simulink model "TWFL_V1"  (R2025b)
settings: Solver=daessc  StartTime=0.0  StopTime=20  RelTol=1e-3
undefined symbols (not defined in the file): dspblkCoreblockFVToolHelper, g, g_fork, g_lift, gcbh, Kd_fork, Kd_lift, Kp_fork, Kp_lift, lx, ly, lz, M, m_w, Mn_33, Mn_44, N, r, T_control, X, Y, Z
libraries: sm_lib x80, nesl_utility x21, simulink x5, slpidlib x1
(part 1 of 3)
settings Model: Creator=oj  LastModifiedBy=itsan
settings DataIOCC: SaveFormat=StructureWithTime
settings OptimizationCC: LifeSpan=inf
settings DebuggingCC: UnconnectedInputMsg=warning  UnconnectedOutputMsg=warning  UnconnectedLineMsg=warning  SFExecutionAtInitializationDiag=none  ArithmeticOperatorsInVariantConditions=warning
settings HardwareCC: ProdBitPerSizeT=32.0  ProdBitPerPtrDiffT=32.0  ProdWordSize=32.0  ProdHWDeviceType=Specified
settings SFSimCC: CustomCodeUndefinedFunction=UseInterfaceOnly
settings RTWCC: GPUComputeCapability=3.5
settings CodeAppCC: StateflowObjectComments=on

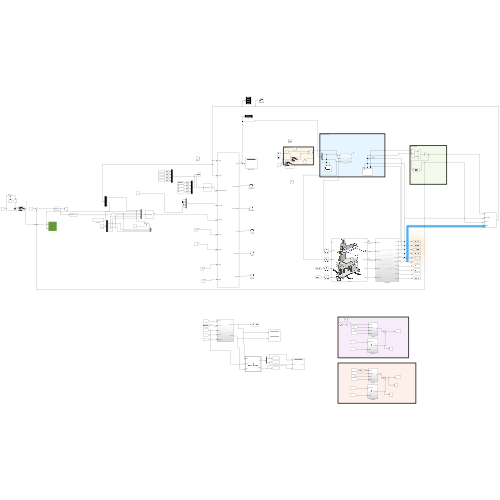
[thumbnail: Simulink's stored preview of the top-level diagram]
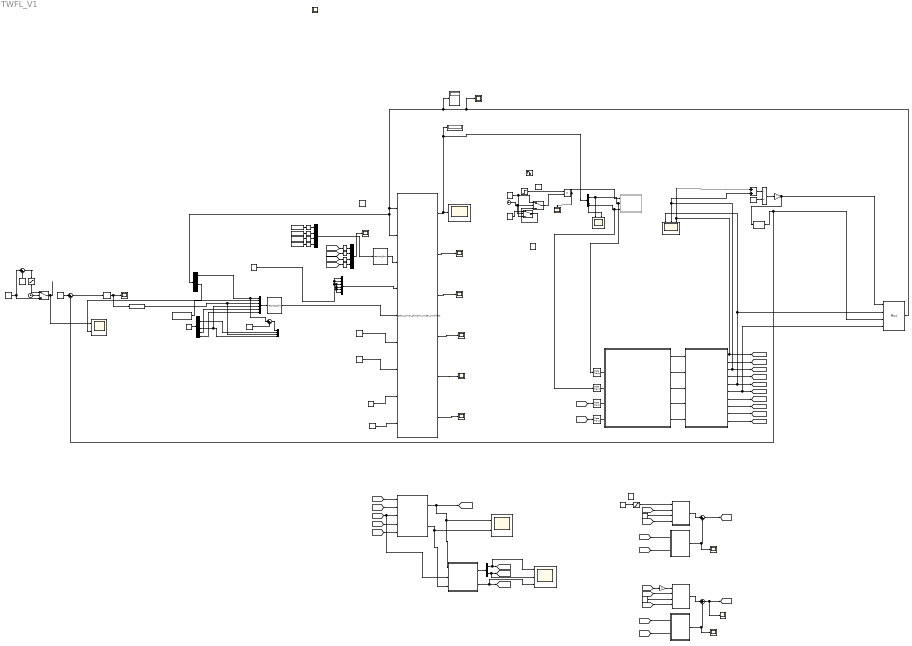
== system TWFL_V1 ==
  note: Simscape model
  note: Calculations
  note: Disturbance
  CPU : Scope
      settings: Description=status  ActiveDisplayYMinimum=-0.000978492283750898  ActiveDisplayYMaximum=0.0013917002145656821  DataLoggingVariableName=ScopeData3
  Calculations : Subsystem
  Clock : Clock
      settings: Decimation=7
  Clock1 : Clock
      settings: Decimation=9
  Constant{,8,13,42..43} (5 alike) : Constant  Value=0
  Constant1 : Constant
  Constant10 : Constant  Value=6
  Constant11 : Constant  Value=-0.1
  Constant12 : Constant  Value=0.8
  Constant14 : Constant  Value=2
  Constant15 : Constant
  Constant2 : Constant  Value=repmat([-50; -pi/4; -3; -pi],N-1,1)
  Constant3 : Constant  Value=repmat([-10;-10],N,1)
  Constant4 : Constant  Value=repmat([500; pi/4; 3; pi],N-1,1)
  Constant45 : Constant  Value=0.0
  Constant5 : Constant
  Constant6 : Constant  Value=2
  Constant7 : Constant  Value=repmat([10;10],N,1)
  Constant9 : Constant  Value=2
  Demux : Demux  Outputs=2
  Demux1 : Demux  Outputs=2
  Demux2 : Demux
  Demux3 : Demux  Outputs=6
  Discrete Derivative : simulink/Discrete/Discrete Derivative  gainval=1.0  ICPrevScaledInput=0.0  OutMin=[]  OutMax=[]  OutDataType=fixdt(1, 16)  OutScaling=2^-10  DoSatur=off
  Display1 : Display
  Divide : Product  Inputs=**
  Divide1 : Product  Inputs=*/
  Fork DOB : Subsystem
  Gain18 : Gain  Gain=-1
  Gain2 : Gain  Gain=r
  KKT residual : Scope
      settings: Description=status  ActiveDisplayYMinimum=-0.32883901659053916  ActiveDisplayYMaximum=1.592767698176573  DataLoggingVariableName=ScopeData4
  Lift DOB : Subsystem
  MATLAB Function1 : MATLAB Function  TreatAsAtomicUnit=on
  Mux{,1,4..5} (4 alike) : Mux
      Mux settings: DisplayOption=signals
  Mux2 : Mux  Inputs=6
  Mux3 : Mux  Inputs=6
  OCP status : Scope
      settings: Description=status  ActiveDisplayYMinimum=-2.0851401210050069  ActiveDisplayYMaximum=5.2280116787993132
  PD fork : Subsystem
  PD lift : Subsystem
  PID Controller : slpidlib/PID Controller  Controller=PID  Form=Parallel  TimeDomain=Discrete-time  UseExternalTs=off  SampleTime=-1  IntegratorMethod=Forward Euler  FilterMethod=Forward Euler  ControllerParametersSource=internal  P=2  I=1  UseKiTs=off  D=0  UseExternalDerivativeSource=off  N=100  UseFilter=on  TunerSelectOption=Transfer Function Based (PID Tuner App)  InitialConditionSource=internal  InitialConditionForIntegrator=0  InitialConditionForFilter=0  DifferentiatorICPrevScaledInput=0  ExternalReset=none  TrackingMode=off  Kt=1  LimitOutput=off  SatLimitsSource=internal  UpperSaturationLimit=inf  LowerSaturationLimit=-inf  LinearizeAsGain=on  AntiWindupMode=none  Kb=1  LimitIntegrator=off  UpperIntegratorSaturationLimit=inf  LowerIntegratorSaturationLimit=-inf  POutMin=[]  POutMax=[]  IOutMin=[]  IOutMax=[]  DOutMin=[]  DOutMax=[]  NOutMin=[]  NOutMax=[]  SumOutMin=[]  SumOutMax=[]  SaturationOutMin=[]  SaturationOutMax=[]  PParamMin=[]  PParamMax=[]  IParamMin=[]  IParamMax=[]  DParamMin=[]  DParamMax=[]  NParamMin=[]  NParamMax=[]  KbParamMin=[]  KbParamMax=[]  KtParamMin=[]  KtParamMax=[]  KbOutMin=[]  KbOutMax=[]  KtOutMin=[]  KtOutMax=[]  IntegratorOutMin=[]  IntegratorOutMax=[]  FilterOutMin=[]  FilterOutMax=[]  SumI1OutMin=[]  SumI1OutMax=[]  SumI2OutMin=[]  SumI2OutMax=[]  SumI3OutMin=[]  SumI3OutMax=[]  SumI4OutMin=[]  SumI4OutMax=[]  SumDOutMin=[]  SumDOutMax=[]  DifferentiatorOutMin=[]  DifferentiatorOutMax=[]  FilterDiffOutCoefMin=[]  FilterDiffOutCoefMax=[]  ReciprocalOutMin=[]  ReciprocalOutMax=[]  SumDenOutMin=[]  SumDenOutMax=[]  SumNumOutMin=[]  SumNumOutMax=[]  DivideOutMin=[]  DivideOutMax=[]  UdiffTsProdOutMin=[]  UdiffTsProdOutMax=[]  NTsProdOutMin=[]  NTsProdOutMax=[]  UintegralTsProdOutMin=[]  UintegralTsProdOutMax=[]  UngainTsProdOutMin=[]  UngainTsProdOutMax=[]  ClampingZeroOutDataTypeStr=Inherit: Inherit via back propagation  ClampingZeroOutMin=[]  ClampingZeroOutMax=[]  FilterDenConstantOutDataTypeStr=Inherit: Inherit via back propagation  FilterDenConstantOutMin=[]  FilterDenConstantOutMax=[]  PCopyOutDataTypeStr=Inherit: Inherit via back propagation  PCopyOutMin=[]  PCopyOutMax=[]  NCopyOutDataTypeStr=Inherit: Inherit via back propagation  NCopyOutMin=[]  NCopyOutMax=[]  IntegratorContinuousStateAttributes=''  IntegratorStateMustResolveToSignalObject=off  IntegratorRTWStateStorageClass=Auto  FilterContinuousStateAttributes=''  FilterStateMustResolveToSignalObject=off  FilterRTWStateStorageClass=Auto  ParallelPVariant=InternalParameters  IdealPVariant=Disabled  IVariant=InternalParameters  DVariant=InternalParameters  IntegratorVariant=Discrete  SatVariant=Disabled  AWVariant=Passthrough  PCopyVariant=Disabled  TRVariant=Disabled  FdbkBlocksVariant=Forward  IdealPFdbkVariant=Disabled  SatFdbkVariant=Disabled  DerivativeFilterVariant=ForwardEulerFilter  NVariant=InternalParameters  NCopyVariant=Disabled  FilterICVariant=InternalICsFilter  IntegratorICVariant=InternalICs  ExternalResetVariant=Disabled  TRSumVariant=Passthrough  SumFdbkVariant=Disabled  SumVariant=Sum_PID  TsampFilterVariant=InternalTs  TsampNgainVariant=Passthrough  TsampIntegralVariant=Disabled_SignalSpec  ExternalSaturationOutDataTypeStr=Inherit: Same as second input  DerivativeSourceVariant=ErrorSignal  PreIntVariant=InternalPreInt
  Plant : Subsystem  Commented=on
  Plant5 : Subsystem
      mask Display: image('plant.png');
  Ramp : simulink/Sources/Ramp  slope=4  start=1  InitialOutput=0
  Ramp1 : simulink/Sources/Ramp  slope=0.05  start=1  InitialOutput=0
  Ramp2 : simulink/Sources/Ramp  slope=1  start=9  InitialOutput=0
  Rate Transition{,1..3} (4 alike) : RateTransition  OutPortSampleTime=T_control
  S-Function : S-Function  FunctionName=repmat_sfun  Parameters=N-1  SFunctionDeploymentMode=off  EnableBusSupport=off
  S-Function1 : S-Function  FunctionName=acados_solver_sfunction_model_simplified  SFunctionDeploymentMode=off  EnableBusSupport=off
      mask Display:
      | % from the make_sfun file
      | global sfun_input_names sfun_output_names
      | for i = 1:length(sfun_input_names)
      | 	port_label('input', i, sfun_input_names{i})
      | end
      | for i = 1:length(sfun_output_names)
      | 	port_label('output', i, sfun_output_names{i})
      | end
  S-Function2 : S-Function  FunctionName=repmat_sfun  Parameters=N+1  SFunctionDeploymentMode=off  EnableBusSupport=off
  SQP iter : Scope
      settings: Description=status  ActiveDisplayYMinimum=0.875  ActiveDisplayYMaximum=2.125  DataLoggingVariableName=ScopeData5
  Saturation : Saturate  UpperLimit=5  LowerLimit=0
  Saturation2 : Saturate  UpperLimit=.25
  Scope control : Scope
      settings: ActiveDisplayYMinimum=-179.76344795838239  ActiveDisplayYMaximum=28.261944980460278  DataLoggingVariableName=ScopeData6
  Scope state : Scope
      settings: ActiveDisplayYMinimum=-0.50123790367694254  ActiveDisplayYMaximum=0.42460054813556447  DataLoggingVariableName=ScopeData7
  Scope2 : Scope  NumInputPorts=3
      settings: ActiveDisplayYMinimum=-0.20198063479091835  ActiveDisplayYMaximum=0.15327811856996762  DataLoggingVariableName=ScopeData9
  Scope26 : Scope  NumInputPorts=2
      settings: ActiveDisplayYMinimum=-5.5444382894798494  ActiveDisplayYMaximum=19.314835391492366  DataLoggingVariableName=ScopeData32
  Scope{,4..5,7,29..31} (7 alike) : Scope
      Scope29 settings: ActiveDisplayYMinimum=-96.648348177302324  ActiveDisplayYMaximum=-32.034536436658129  DataLoggingVariableName=ScopeData36
      Scope30 settings: ActiveDisplayYMinimum=-184.47481197821281  ActiveDisplayYMaximum=541.97444620327656  DataLoggingVariableName=ScopeData35
      Scope31 settings: ActiveDisplayYMinimum=-107.02501908705908  ActiveDisplayYMaximum=9.012103475779579  DataLoggingVariableName=ScopeData37
      Scope4 settings: ActiveDisplayYMinimum=-15.603117153759081  ActiveDisplayYMaximum=28.598103704711281  DataLoggingVariableName=ScopeData11
      Scope5 settings: ActiveDisplayYMinimum=-0.32762488910758569  ActiveDisplayYMaximum=3.4436733955388874  DataLoggingVariableName=ScopeData12
      Scope7 settings: ActiveDisplayYMinimum=-0.36432624038755357  ActiveDisplayYMaximum=6.747864665777934  DataLoggingVariableName=ScopeData19
      Scope settings: ActiveDisplayYMinimum=-13.79726  ActiveDisplayYMaximum=10.28583
  Scope3 : Scope  NumInputPorts=2
      settings: ActiveDisplayYMinimum=-0.28208251457945138  ActiveDisplayYMaximum=0.11496904410617963  DataLoggingVariableName=ScopeData10
  Scope6 : Scope  NumInputPorts=2
      settings: ActiveDisplayYMinimum=-1.0752841178040073  ActiveDisplayYMaximum=3.1865041498100037  DataLoggingVariableName=ScopeData13
  Scope8 : Scope  NumInputPorts=3
      settings: ActiveDisplayYMinimum=-5.0680991382670406  ActiveDisplayYMaximum=15.726284673069914  DataLoggingVariableName=ScopeData21
  Signal Specification : SignalSpecification  OutDataTypeStr=double  Dimensions=1
  Signal Specification{1..8} (8 alike) : SignalSpecification  Dimensions=1
  Sine Wave : Sin  Frequency=6*pi  SampleTime=0
  Step : Step  After=30  SampleTime=0
  Subsystem : Subsystem
  Sum : Sum  Inputs=+|+
  Sum16 : Sum  Inputs=|++
  Sum17 : Sum  Inputs=|++
  Sum3 : Sum  Inputs=|+-
  Sum4 : Sum  Inputs=|++
  Sum5 : Sum  Inputs=|+-
  Switch : Switch  Criteria=u2 > Threshold  Threshold=4  SaturateOnIntegerOverflow=off  InputSameDT=off
  Switch1 : Switch  Criteria=u2 > Threshold  Threshold=3  SaturateOnIntegerOverflow=off  InputSameDT=off
  Switch2 : Switch  Criteria=u2 > Threshold  SaturateOnIntegerOverflow=off  InputSameDT=off
  ref pitch : Constant  Value=0.0535
  u : Display
  weights : Constant  Value=repmat([5;3;0;1e-3], 244/4, 1)
  x1 ocp : Scope
      settings: Description=status  ActiveDisplayYMinimum=-2.6422889921421415  ActiveDisplayYMaximum=2.2266101006407979  DataLoggingVariableName=ScopeData2
  y_ref4 : Constant  Value=[1; 0; 0; 0; 0; 0]
  wires:
  S-Function1/5 -> CPU/1
  S-Function1/6 -> SQP iter/1
  S-Function1/3 -> KKT residual/1
  Mux/1 -> Display1/1, Demux2/1, S-Function1/2, S-Function1/1, Scope state/1  "x"
  S-Function1/4 -> x1 ocp/1
  S-Function1/2 -> OCP status/1
  Clock/1 -> Switch1/2, Switch/2
  Constant/1 -> Switch1/3, Switch/1
  Divide/1 -> Scope5/1, Plant/1(dF)
  Switch/1 -> Divide/2
  S-Function1/1 -> u/1, Demux/1, Scope control/1  "u"
  Switch1/1 -> Switch/3
  Constant1/1 -> Switch1/1
  Constant2/1 -> S-Function1/6
  Mux3/1 -> S-Function1/4
  Demux/1 -> Scope3/1, Rate Transition2/1, Plant/2(rwTorque)
  Calculations/1(rw_pos) -> Sum/1, Scope2/3, [rw_pos]  "rw_angle"
  Calculations/3(lw_pos) -> Sum/2, Scope2/2, [lw_pos]  "lw_angle"
  Calculations/5(pitch_pos) -> Mux/2, Scope2/1, [pitch_pos]  "pitch_angle"
  Sum/1 -> Divide1/1
  Constant6/1 -> Divide1/2
  Divide1/1 -> Gain2/1
  Gain2/1 -> Discrete Derivative/1, Mux/1  "x"
  Discrete Derivative/1 -> Mux/3, Sum3/2  "x_dot"
  Constant3/1 -> S-Function1/8
  Constant7/1 -> S-Function1/9
  Step/1 -> Divide/1
  Demux/2 -> Rate Transition3/1, Plant/3(lwTorque), Scope3/2
  S-Function/1 -> S-Function1/5
  Mux2/1 -> S-Function/1
  y_ref4/1 -> Demux3/1
  Demux3/4 -> Mux2/4, Mux1/4
  Demux3/6 -> Mux2/6
  Demux3/5 -> Mux2/5
  Demux2/1 -> Sum4/1, Mux2/1
  Sum3/1 -> PID Controller/1
  Constant13/1 -> Mux3/1, Mux3/2, Mux3/6, Mux3/5, Mux3/4, Mux3/3
  Constant14/1 -> Switch2/3, Sum5/1
  PID Controller/1 -> Signal Specification/1, Scope4/1
  Signal Specification/1 -> Mux2/3, Mux1/3
  Demux3/2 -> Mux1/2
  Sum4/1 -> Mux1/1
  Constant15/1 -> Sum4/2
  Constant4/1 -> S-Function1/7
  Ramp2/1 -> Sum5/2
  Clock1/1 -> Switch2/2
  Sum5/1 -> Saturation/1
  Saturation/1 -> Switch2/1
  Switch2/1 -> Scope6/1  "reference_v"
  Demux2/3 -> Scope6/2
  ref pitch/1 -> Mux2/2
  Calculations/4(lw_vel) -> [lw_vel]
  Calculations/9(arm_pos) -> [arm_pos]
  Calculations/8(lift_vel) -> [lift_vel]
  Plant5/5(armPos) -> Calculations/5(arm_angle)
  Plant5/4(lift_pos) -> Calculations/4(lift_height)
  Calculations/7(lift_pos) -> [lift_pos]
  Rate Transition1/1 -> Plant5/4(liftForce)
  [force_lift] -> Rate Transition1/1
  [arm_pos] -> Subsystem/4(arm_pos)
  Rate Transition/1 -> Plant5/5(armTorque)
  Plant5/3(pitch_angle) -> Calculations/3(pitch_angle)  "pitch_angle"
  Calculations/6(pitch_vel) -> Mux/4, [pitch_vel]
  Plant5/1(rw_angle) -> Calculations/1(rw_angle)  "rw_angle"
  [force_lift] -> Subsystem/1(force_lift)
  Plant5/2(lw_angle) -> Calculations/2(lw_angle)  "lw_angle"
  [lift_pos] -> MATLAB Function1/2(pos_lift), Subsystem/3(lift_pos)
  Subsystem/1(mass_hat) -> [mass_hat], MATLAB Function1/1(m_hat), Scope26/1
  Calculations/2(rw_vel) -> [rw_vel]
  [torque_arm] -> Subsystem/5(torque_arm)
  [pitch_pos] -> Subsystem/2(pitch_pos)
  Calculations/10(arm_vel) -> [arm_vel]
  [torque_arm] -> Rate Transition/1
  Rate Transition2/1 -> Plant5/2(rwTorque)
  Rate Transition3/1 -> Plant5/3(lwTorque)
  Constant8/1 -> Sum3/1
  MATLAB Function1/1(cdg) -> Demux1/1
  Demux1/1 -> Scope8/1, [cog_x]
  Demux1/2 -> Scope8/2, [cog_z]
  MATLAB Function1/2(I_total) -> Scope8/3, [inertia]
  [mass_hat] -> Signal Specification4/1
  [inertia] -> Signal Specification3/1
  [cog_x] -> Signal Specification2/1
  [cog_z] -> Signal Specification1/1
  Signal Specification1/1 -> Mux4/4
  Signal Specification2/1 -> Mux4/3
  Signal Specification3/1 -> Mux4/2
  Signal Specification4/1 -> Mux4/1
  Subsystem/2(dist_hat) -> MATLAB Function1/3(d_hat), Scope26/2
  Sum17/1 -> [force_lift]
  [pitch_pos] -> Gain18/1
  [lift_pos] -> PD lift/2(posMeas)
  [force_lift] -> Lift DOB/1(Input Torque)
  Constant42/1 -> PD fork/3(velRef)
  Constant43/1 -> PD lift/3(velRef)
  Fork DOB/1(Est_dis) -> Scope29/1, Sum16/2
  Lift DOB/1(Est_dis) -> Sum17/2, Scope30/1
  [lift_vel] -> PD lift/4(velMeas)
  [torque_arm] -> Fork DOB/1(Input Torque)
  Sum16/1 -> Scope31/1, [torque_arm]
  PD lift/1(out) -> Sum17/1
  Ramp1/1 -> Saturation2/1
  [arm_vel] -> Fork DOB/2(Velocity)
  PD fork/1(out) -> Sum16/1
  Gain18/1 -> PD fork/1(posRef)
  [arm_vel] -> PD fork/4(velMeas)
  [lift_vel] -> Lift DOB/2(Velocity)
  [arm_pos] -> PD fork/2(posMeas)
  Mux4/1 -> Scope7/1
  S-Function2/1 -> S-Function1/3
  Signal Specification8/1 -> Mux5/1
  Signal Specification7/1 -> Mux5/2
  Signal Specification6/1 -> Mux5/3
  Signal Specification5/1 -> Mux5/4
  Constant12/1 -> Signal Specification5/1
  Constant11/1 -> Signal Specification6/1
  Constant10/1 -> Signal Specification7/1
  Constant9/1 -> Signal Specification8/1
  Mux5/1 -> S-Function2/1
  Saturation2/1 -> PD lift/1(posRef)

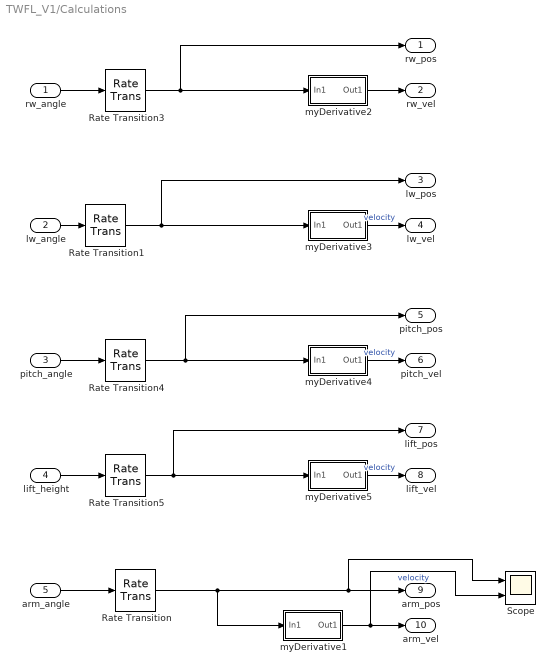
== system TWFL_V1/Calculations ==
  rw_angle : Inport
  lw_angle : Inport  Port=2
  pitch_angle : Inport  Port=3
  lift_height : Inport  Port=4
  arm_angle : Inport  Port=5
  Rate Transition{,1,3..5} (5 alike) : RateTransition  OutPortSampleTime=T_control
  Scope : Scope  NumInputPorts=2
      settings: ActiveDisplayYMinimum=-0.3840409140605956  ActiveDisplayYMaximum=2.1541582270060031  DataLoggingVariableName=ScopeData22
  myDerivative1 : Subsystem
      mask Display: image('myDerivative.png');
  myDerivative2 : Subsystem
      mask Display: image('myDerivative.png');
  myDerivative3 : Subsystem
      mask Display: image('myDerivative.png');
  myDerivative4 : Subsystem
      mask Display: image('myDerivative.png');
  myDerivative5 : Subsystem
      mask Display: image('myDerivative.png');
  rw_pos : Outport
  rw_vel : Outport  Port=2
  lw_pos : Outport  Port=3
  lw_vel : Outport  Port=4
  pitch_pos : Outport  Port=5
  pitch_vel : Outport  Port=6
  lift_pos : Outport  Port=7
  lift_vel : Outport  Port=8
  arm_pos : Outport  Port=9
  arm_vel : Outport  Port=10
  wires:
  rw_angle/1 -> Rate Transition3/1
  lw_angle/1 -> Rate Transition1/1
  pitch_angle/1 -> Rate Transition4/1
  Rate Transition5/1 -> myDerivative5/1(In1), lift_pos/1
  myDerivative2/1(Out1) -> rw_vel/1
  myDerivative3/1(Out1) -> lw_vel/1  "velocity"
  myDerivative4/1(Out1) -> pitch_vel/1  "velocity"
  myDerivative5/1(Out1) -> lift_vel/1  "velocity"
  lift_height/1 -> Rate Transition5/1
  arm_angle/1 -> Rate Transition/1
  myDerivative1/1(Out1) -> Scope/2, arm_vel/1  "velocity"
  Rate Transition/1 -> myDerivative1/1(In1), Scope/1, arm_pos/1
  Rate Transition1/1 -> myDerivative3/1(In1), lw_pos/1
  Rate Transition3/1 -> myDerivative2/1(In1), rw_pos/1
  Rate Transition4/1 -> myDerivative4/1(In1), pitch_pos/1

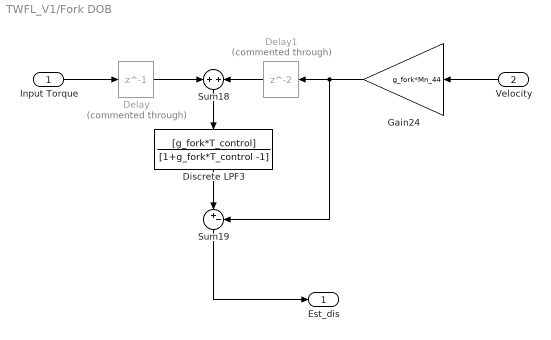
== system TWFL_V1/Fork DOB ==
  Input Torque : Inport
  Velocity : Inport  Port=2
  Delay : Delay  Commented=through  DelayLength=1  InputProcessing=Columns as channels (frame based)  SampleTime=T_control
  Delay1 : Delay  Commented=through  InputProcessing=Columns as channels (frame based)  SampleTime=T_control
  Discrete LPF3 : DiscreteFilter  LoadFcn=dspblkCoreblockFVToolHelper(gcbh,'load');  Numerator=[g_fork*T_control]  Denominator=[1+g_fork*T_control -1]
      settings: CopyFcn=dspblkCoreblockFVToolHelper(gcbh,'copy');  DeleteFcn=dspblkCoreblockFVToolHelper(gcbh,'close');  ModelCloseFcn=dspblkCoreblockFVToolHelper(gcbh,'close');  PreSaveFcn=dspblkCoreblockFVToolHelper(gcbh,'presave');  PostSaveFcn=dspblkCoreblockFVToolHelper(gcbh,'postsave');  CloseFcn=dspblkCoreblockFVToolHelper(gcbh,'close');
  Gain24 : Gain  Gain=g_fork*Mn_44
  Sum18 : Sum  Inputs=+|+
  Sum19 : Sum  Inputs=|+-
  Est_dis : Outport
  wires:
  Delay/1 -> Sum18/1
  Sum19/1 -> Est_dis/1
  Velocity/1 -> Gain24/1
  Input Torque/1 -> Delay/1
  Sum18/1 -> Discrete LPF3/1
  Gain24/1 -> Sum19/2, Delay1/1
  Discrete LPF3/1 -> Sum19/1
  Delay1/1 -> Sum18/2

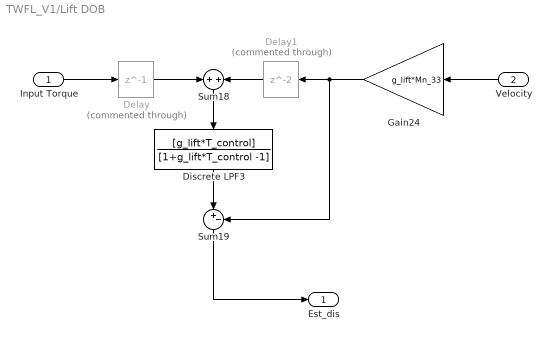
== system TWFL_V1/Lift DOB ==
  Input Torque : Inport
  Velocity : Inport  Port=2
  Delay : Delay  Commented=through  DelayLength=1  InputProcessing=Columns as channels (frame based)  SampleTime=T_control
  Delay1 : Delay  Commented=through  InputProcessing=Columns as channels (frame based)  SampleTime=T_control
  Discrete LPF3 : DiscreteFilter  LoadFcn=dspblkCoreblockFVToolHelper(gcbh,'load');  Numerator=[g_lift*T_control]  Denominator=[1+g_lift*T_control -1]
      settings: CopyFcn=dspblkCoreblockFVToolHelper(gcbh,'copy');  DeleteFcn=dspblkCoreblockFVToolHelper(gcbh,'close');  ModelCloseFcn=dspblkCoreblockFVToolHelper(gcbh,'close');  PreSaveFcn=dspblkCoreblockFVToolHelper(gcbh,'presave');  PostSaveFcn=dspblkCoreblockFVToolHelper(gcbh,'postsave');  CloseFcn=dspblkCoreblockFVToolHelper(gcbh,'close');
  Gain24 : Gain  Gain=g_lift*Mn_33
  Sum18 : Sum  Inputs=+|+
  Sum19 : Sum  Inputs=|+-
  Est_dis : Outport
  wires:
  Delay1/1 -> Sum18/2
  Discrete LPF3/1 -> Sum19/1
  Gain24/1 -> Delay1/1, Sum19/2
  Sum18/1 -> Discrete LPF3/1
  Input Torque/1 -> Delay/1
  Velocity/1 -> Gain24/1
  Sum19/1 -> Est_dis/1
  Delay/1 -> Sum18/1

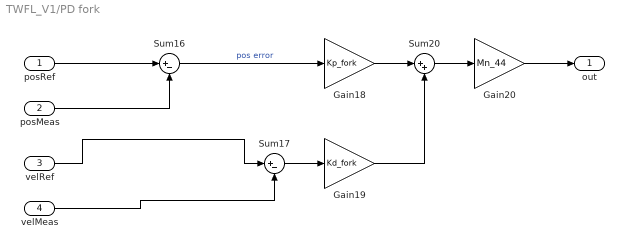
== system TWFL_V1/PD fork ==
  posRef : Inport
  posMeas : Inport  Port=2
  velRef : Inport  Port=3
  velMeas : Inport  Port=4
  Gain18 : Gain  Gain=Kp_fork
  Gain19 : Gain  Gain=Kd_fork
  Gain20 : Gain  Gain=Mn_44
  Sum16 : Sum  Inputs=|+-
  Sum17 : Sum  Inputs=|+-
  Sum20 : Sum  Inputs=|++
  out : Outport
  wires:
  Sum16/1 -> Gain18/1  "pos error"
  Gain18/1 -> Sum20/1
  Sum17/1 -> Gain19/1
  posRef/1 -> Sum16/1
  Sum20/1 -> Gain20/1
  Gain19/1 -> Sum20/2
  Gain20/1 -> out/1
  posMeas/1 -> Sum16/2
  velRef/1 -> Sum17/1
  velMeas/1 -> Sum17/2

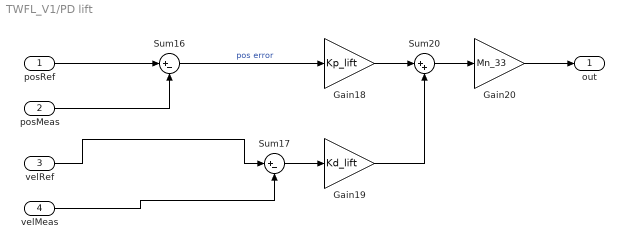
== system TWFL_V1/PD lift ==
  posRef : Inport
  posMeas : Inport  Port=2
  velRef : Inport  Port=3
  velMeas : Inport  Port=4
  Gain18 : Gain  Gain=Kp_lift
  Gain19 : Gain  Gain=Kd_lift
  Gain20 : Gain  Gain=Mn_33
  Sum16 : Sum  Inputs=|+-
  Sum17 : Sum  Inputs=|+-
  Sum20 : Sum  Inputs=|++
  out : Outport
  wires:
  velMeas/1 -> Sum17/2
  velRef/1 -> Sum17/1
  posMeas/1 -> Sum16/2
  Gain20/1 -> out/1
  Gain19/1 -> Sum20/2
  Sum20/1 -> Gain20/1
  posRef/1 -> Sum16/1
  Sum17/1 -> Gain19/1
  Gain18/1 -> Sum20/1
  Sum16/1 -> Gain18/1  "pos error"

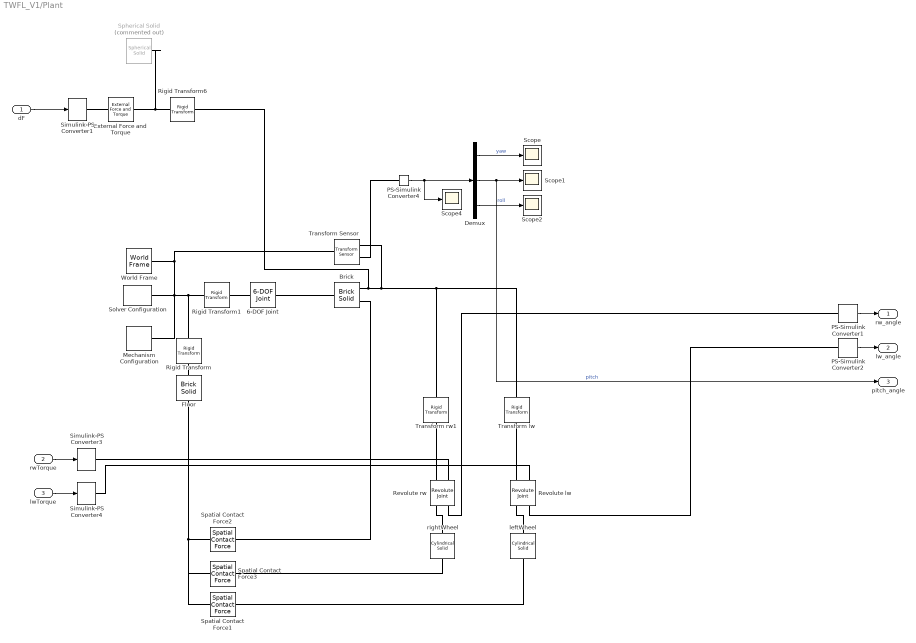
== system TWFL_V1/Plant ==
  dF : Inport
  rwTorque : Inport  Port=2
  lwTorque : Inport  Port=3
  6-DOF Joint : sm_lib/Joints/6-DOF Joint  JointMode=Normal  CompositeWrenchDir=BaseOnFollower  CompositeWrenchFrame=BaseFrame  SenseConstraintForce=off  SenseConstraintTorque=off  SenseTotalForce=off  SenseTotalTorque=off  PxPositionTargetSpecify=off  PxPositionTargetPriority=High  PxPositionTargetValue=0  PxPositionTargetValueUnits=m  PxVelocityTargetSpecify=off  PxVelocityTargetPriority=High  PxVelocityTargetValue=0  PxVelocityTargetValueUnits=m/s  PxEquilibriumPosition=0  PxEquilibriumPositionUnits=m  PxSpringStiffness=0  PxSpringStiffnessUnits=N/m  PxDampingCoefficient=0  PxDampingCoefficientUnits=N/(m/s)  PxLowerLimitSpecify=off  PxLowerLimitBound=-1  PxLowerLimitBoundUnits=m  PxLowerLimitStiffness=1e6  PxLowerLimitStiffnessUnits=N/m  PxLowerLimitDamping=1e3  PxLowerLimitDampingUnits=N/(m/s)  PxLowerLimitTransitionRegionWidth=1e-4  PxLowerLimitTransitionRegionWidthUnits=m  PxUpperLimitSpecify=off  PxUpperLimitBound=1  PxUpperLimitBoundUnits=m  PxUpperLimitStiffness=1e6  PxUpperLimitStiffnessUnits=N/m  PxUpperLimitDamping=1e3  PxUpperLimitDampingUnits=N/(m/s)  PxUpperLimitTransitionRegionWidth=1e-4  PxUpperLimitTransitionRegionWidthUnits=m  PxTorqueActuationMode=NoTorque  PxMotionActuationMode=ComputedMotion  PxSensePosition=off  PxSenseVelocity=off  PxSenseAcceleration=off  PxSenseTorqueForce=off  PxSenseLowerLimitTorqueForce=off  PxSenseUpperLimitTorqueForce=off  PyPositionTargetSpecify=off  PyPositionTargetPriority=High  PyPositionTargetValue=0  PyPositionTargetValueUnits=m  PyVelocityTargetSpecify=off  PyVelocityTargetPriority=High  PyVelocityTargetValue=0  PyVelocityTargetValueUnits=m/s  PyEquilibriumPosition=0  PyEquilibriumPositionUnits=m  PySpringStiffness=0  PySpringStiffnessUnits=N/m  PyDampingCoefficient=0  PyDampingCoefficientUnits=N/(m/s)  PyLowerLimitSpecify=off  PyLowerLimitBound=-1  PyLowerLimitBoundUnits=m  PyLowerLimitStiffness=1e6  PyLowerLimitStiffnessUnits=N/m  PyLowerLimitDamping=1e3  PyLowerLimitDampingUnits=N/(m/s)  PyLowerLimitTransitionRegionWidth=1e-4  PyLowerLimitTransitionRegionWidthUnits=m  PyUpperLimitSpecify=off  PyUpperLimitBound=1  PyUpperLimitBoundUnits=m  PyUpperLimitStiffness=1e6  PyUpperLimitStiffnessUnits=N/m  PyUpperLimitDamping=1e3  PyUpperLimitDampingUnits=N/(m/s)  PyUpperLimitTransitionRegionWidth=1e-4  PyUpperLimitTransitionRegionWidthUnits=m  PyTorqueActuationMode=NoTorque  PyMotionActuationMode=ComputedMotion  PySensePosition=off  PySenseVelocity=off  PySenseAcceleration=off  PySenseTorqueForce=off  PySenseLowerLimitTorqueForce=off  PySenseUpperLimitTorqueForce=off  PzPositionTargetSpecify=off  PzPositionTargetPriority=High  PzPositionTargetValue=0  PzPositionTargetValueUnits=m  PzVelocityTargetSpecify=off  PzVelocityTargetPriority=High  PzVelocityTargetValue=0  PzVelocityTargetValueUnits=m/s  PzEquilibriumPosition=0  PzEquilibriumPositionUnits=m  PzSpringStiffness=0  PzSpringStiffnessUnits=N/m  PzDampingCoefficient=0  PzDampingCoefficientUnits=N/(m/s)  PzLowerLimitSpecify=off  PzLowerLimitBound=-1  PzLowerLimitBoundUnits=m  PzLowerLimitStiffness=1e6  PzLowerLimitStiffnessUnits=N/m  PzLowerLimitDamping=1e3  PzLowerLimitDampingUnits=N/(m/s)  PzLowerLimitTransitionRegionWidth=1e-4  PzLowerLimitTransitionRegionWidthUnits=m  PzUpperLimitSpecify=off  PzUpperLimitBound=1  PzUpperLimitBoundUnits=m  PzUpperLimitStiffness=1e6  PzUpperLimitStiffnessUnits=N/m  PzUpperLimitDamping=1e3  PzUpperLimitDampingUnits=N/(m/s)  PzUpperLimitTransitionRegionWidth=1e-4  PzUpperLimitTransitionRegionWidthUnits=m  PzTorqueActuationMode=NoTorque  PzMotionActuationMode=ComputedMotion  PzSensePosition=off  PzSenseVelocity=off  PzSenseAcceleration=off  PzSenseTorqueForce=off  PzSenseLowerLimitTorqueForce=off  PzSenseUpperLimitTorqueForce=off  SphPositionTargetSpecify=off  SphPositionTargetPriority=High  SphPositionTargetRotationMethod=None  SphPositionTargetFollAlignAxisA=+X  SphPositionTargetBaseAlignAxisA=+Y  SphPositionTargetFollAlignAxisB=+Y  SphPositionTargetBaseAlignAxisB=+Z  SphPositionTargetRotationStandardAxis=+Z  SphPositionTargetRotationAngle=0  SphPositionTargetRotationAngleUnits=deg  SphPositionTargetRotationArbitraryAxis=[0 0 1]  SphPositionTargetRotationSequenceAxes=FollowerAxes  SphPositionTargetRotationSequence=XYX  SphPositionTargetRotationSequenceAngles=[0 0 0]  SphPositionTargetRotationSequenceAnglesUnits=deg  SphPositionTargetRotationMatrix=[1 0 0;0 1 0;0 0 1]  SphPositionTargetQuaternion=[1 0 0 0]  SphVelocityTargetSpecify=off  SphVelocityTargetPriority=High  SphVelocityTargetValue=[0 0 0]  SphVelocityTargetValueUnits=deg/s  SphVelocityTargetInFollowerFrame=on  SphEqPosRotationMethod=None  SphEqPosFollAlignAxisA=+X  SphEqPosBaseAlignAxisA=+Y  SphEqPosFollAlignAxisB=+Y  SphEqPosBaseAlignAxisB=+Z  SphEqPosRotationStandardAxis=+Z  SphEqPosRotationAngle=0  SphEqPosRotationAngleUnits=deg  SphEqPosRotationArbitraryAxis=[0 0 1]  SphEqPosRotationSequenceAxes=FollowerAxes  SphEqPosRotationSequence=XYX  SphEqPosRotationSequenceAngles=[0 0 0]  SphEqPosRotationSequenceAnglesUnits=deg  SphEqPosRotationMatrix=[1 0 0;0 1 0;0 0 1]  SphEqPosQuaternion=[1 0 0 0]  SphSpringStiffness=0  SphSpringStiffnessUnits=N*m/deg  SphDampingCoefficient=0  SphDampingCoefficientUnits=N*m/(deg/s)  SphLowerLimitSpecify=off  SphLowerLimitBound=15  SphLowerLimitBoundUnits=deg  SphLowerLimitStiffness=1e4  SphLowerLimitStiffnessUnits=N*m/deg  SphLowerLimitDamping=10  SphLowerLimitDampingUnits=N*m/(deg/s)  SphLowerLimitTransitionRegionWidth=0.1  SphLowerLimitTransitionRegionWidthUnits=deg  SphUpperLimitSpecify=off  SphUpperLimitBound=45  SphUpperLimitBoundUnits=deg  SphUpperLimitStiffness=1e4  SphUpperLimitStiffnessUnits=N*m/deg  SphUpperLimitDamping=10  SphUpperLimitDampingUnits=N*m/(deg/s)  SphUpperLimitTransitionRegionWidth=0.1  SphUpperLimitTransitionRegionWidthUnits=deg  SphTorqueActuationMode=NoTorque  SphActuateTorqueX=off  SphActuateTorqueY=off  SphActuateTorqueZ=off  SphActuateTorque=off  SphActuationFrame=BaseFrame  SphSensePosition=off  SphSenseVelocityX=off  SphSenseVelocityY=off  SphSenseVelocityZ=off  SphSenseVelocity=off  SphSenseAccelerationX=off  SphSenseAccelerationY=off  SphSenseAccelerationZ=off  SphSenseAcceleration=off  SphSenseLowerLimitTorqueMag=off  SphSenseUpperLimitTorqueMag=off  SphSensingFrame=BaseFrame
  Brick : sm_lib/Body Elements/Brick Solid  BrickDimensions=[lx ly lz]  BrickDimensionsUnits=m  ExportEntireGeometry=on  InertiaType=CalculateFromGeometry  BasedOnType=Mass  Density=1000  DensityUnits=kg/(m^3)  Mass=M  MassUnits=kg  CenterOfMass=[0 0 0]  CenterOfMassUnits=m  MomentsOfInertia=[1 1 1]  MomentsOfInertiaUnits=kg*m^2  ProductsOfInertia=[0 0 0]  ProductsOfInertiaUnits=kg*m^2  GraphicType=FromGeometry  MarkerShape=Sphere  MarkerSize=10  GraphicVisPropType=SimpleVisualProperties  GraphicDiffuseColor=[0.8 0.0 0.2]  GraphicOpacity=0.6  GraphicSpecularColor=[0.5 0.5 0.5 1.0]  GraphicAmbientColor=[0.15 0.15 0.15 1.0]  GraphicEmissiveColor=[0.0 0.0 0.0 1.0]  GraphicShininess=75  DoExposeReferenceFrame=on  SerializedFrames=|
      | <Frames>
      | 
      |   <Frame>
      |     <Id>Frame2</Id>
      |     <Value>
      |       <Name>B</Name>
      |       <Origin>
      |         <Source>GeometricFeature</Source>
      |         <FeatureName>-z surface</FeatureName>
      |       </Origin>
      |       <PrimaryAxis>
      |         <DefinedDirection>+Z</DefinedDirection>
      |         <Source>ReferenceFrame</Source>
      |         <SourceDirection>+Z</SourceDirection>
      |         <FeatureName></FeatureName>
      |       </PrimaryAxis>
      |       <SecondaryAxis>
      |         <DefinedDirection>+X</DefinedDirection>
      |         <Source>ReferenceFrame</Source>
      |         <SourceDirection>+X</SourceDirection>
      |         <FeatureName></FeatureName>
      |       </SecondaryAxis>
      |     </Value>
      |   </Frame>
      | 
      | </Frames>
  Demux : Demux  Outputs=3
  External Force and Torque : sm_lib/Forces and Torques/External Force and Torque  EnableForceX=on  EnableForceY=off  EnableForceZ=off  EnableForce=off  ForceResolutionFrame=World  EnableTorqueX=off  EnableTorqueY=off  EnableTorqueZ=off  EnableTorque=off  TorqueResolutionFrame=AttachedFrame
  Floor : sm_lib/Body Elements/Brick Solid  BrickDimensions=[100 100 0.010]  BrickDimensionsUnits=m  ExportEntireGeometry=on  InertiaType=CalculateFromGeometry  BasedOnType=Density  Density=1000  DensityUnits=kg/m^3  Mass=1  MassUnits=kg  CenterOfMass=[0 0 0]  CenterOfMassUnits=m  MomentsOfInertia=[1 1 1]  MomentsOfInertiaUnits=kg*m^2  ProductsOfInertia=[0 0 0]  ProductsOfInertiaUnits=kg*m^2  GraphicType=FromGeometry  MarkerShape=Sphere  MarkerSize=10  GraphicVisPropType=SimpleVisualProperties  GraphicDiffuseColor=[0.298 0.502 0.1294]  GraphicOpacity=1  GraphicSpecularColor=[0.5 0.5 0.5 1.0]  GraphicAmbientColor=[0.15 0.15 0.15 1.0]  GraphicEmissiveColor=[0.0 0.0 0.0 1.0]  GraphicShininess=75  DoExposeReferenceFrame=on  SerializedFrames=<Frames/>
  Mechanism Configuration : sm_lib/Utilities/Mechanism Configuration  UniformGravity=Constant  GravityVector=[0 0 -9.81]  GravityVectorUnits=m/s^2  LinearizationDelta=0.001  JointModeTransitionNonlinearIterations=2
  PS-Simulink Converter1 : nesl_utility/PS-Simulink Converter  PhysicalDomain=network_engine_domain  SubClassName=ps_output  LeftPortType=input  RightPortType=output  PseudoPeriodic=off  Frequencies=[]  VectorFormat=1-D array  Unit=1  AffineConversion=off
  PS-Simulink Converter2 : nesl_utility/PS-Simulink Converter  PhysicalDomain=network_engine_domain  SubClassName=ps_output  LeftPortType=input  RightPortType=output  PseudoPeriodic=off  Frequencies=[]  VectorFormat=1-D array  Unit=1  AffineConversion=off
  PS-Simulink Converter4 : nesl_utility/PS-Simulink Converter  PhysicalDomain=network_engine_domain  SubClassName=ps_output  LeftPortType=input  RightPortType=output  PseudoPeriodic=off  Frequencies=[]  VectorFormat=inherit  Unit=inherit  AffineConversion=off
  Revolute lw : sm_lib/Joints/Revolute Joint  JointMode=Normal  CompositeWrenchDir=FollowerOnBase  CompositeWrenchFrame=BaseFrame  SenseConstraintForce=off  SenseConstraintTorque=off  SenseTotalForce=off  SenseTotalTorque=off  PositionTargetSpecify=off  PositionTargetPriority=High  PositionTargetValue=0  PositionTargetValueUnits=deg  VelocityTargetSpecify=off  VelocityTargetPriority=High  VelocityTargetValue=0  VelocityTargetValueUnits=deg/s  EquilibriumPosition=0  EquilibriumPositionUnits=deg  SpringStiffness=0  SpringStiffnessUnits=N*m/deg  DampingCoefficient=0  DampingCoefficientUnits=N*m/(deg/s)  LowerLimitSpecify=off  LowerLimitBound=-90  LowerLimitBoundUnits=deg  LowerLimitStiffness=1e4  LowerLimitStiffnessUnits=N*m/deg  LowerLimitDamping=10  LowerLimitDampingUnits=N*m/(deg/s)  LowerLimitTransitionRegionWidth=0.1  LowerLimitTransitionRegionWidthUnits=deg  UpperLimitSpecify=off  UpperLimitBound=90  UpperLimitBoundUnits=deg  UpperLimitStiffness=1e4  UpperLimitStiffnessUnits=N*m/deg  UpperLimitDamping=10  UpperLimitDampingUnits=N*m/(deg/s)  UpperLimitTransitionRegionWidth=0.1  UpperLimitTransitionRegionWidthUnits=deg  TorqueActuationMode=InputTorque  MotionActuationMode=ComputedMotion  SensePosition=on  SenseVelocity=off  SenseAcceleration=off  SenseTorqueForce=off  SenseLowerLimitTorqueForce=off  SenseUpperLimitTorqueForce=off
  Revolute rw : sm_lib/Joints/Revolute Joint  JointMode=Normal  CompositeWrenchDir=FollowerOnBase  CompositeWrenchFrame=BaseFrame  SenseConstraintForce=off  SenseConstraintTorque=off  SenseTotalForce=off  SenseTotalTorque=off  PositionTargetSpecify=off  PositionTargetPriority=High  PositionTargetValue=0  PositionTargetValueUnits=deg  VelocityTargetSpecify=off  VelocityTargetPriority=High  VelocityTargetValue=0  VelocityTargetValueUnits=deg/s  EquilibriumPosition=0  EquilibriumPositionUnits=deg  SpringStiffness=0  SpringStiffnessUnits=N*m/deg  DampingCoefficient=0  DampingCoefficientUnits=N*m/(deg/s)  LowerLimitSpecify=off  LowerLimitBound=-90  LowerLimitBoundUnits=deg  LowerLimitStiffness=1e4  LowerLimitStiffnessUnits=N*m/deg  LowerLimitDamping=10  LowerLimitDampingUnits=N*m/(deg/s)  LowerLimitTransitionRegionWidth=0.1  LowerLimitTransitionRegionWidthUnits=deg  UpperLimitSpecify=off  UpperLimitBound=90  UpperLimitBoundUnits=deg  UpperLimitStiffness=1e4  UpperLimitStiffnessUnits=N*m/deg  UpperLimitDamping=10  UpperLimitDampingUnits=N*m/(deg/s)  UpperLimitTransitionRegionWidth=0.1  UpperLimitTransitionRegionWidthUnits=deg  TorqueActuationMode=InputTorque  MotionActuationMode=ComputedMotion  SensePosition=on  SenseVelocity=off  SenseAcceleration=off  SenseTorqueForce=off  SenseLowerLimitTorqueForce=off  SenseUpperLimitTorqueForce=off
  Rigid Transform : sm_lib/Frames and Transforms/Rigid Transform  RotationMethod=None  FollAlignAxisA=+X  BaseAlignAxisA=+Y  FollAlignAxisB=+Y  BaseAlignAxisB=+Z  RotationStandardAxis=+Z  RotationAngle=0  RotationAngleUnits=deg  RotationArbitraryAxis=[0 0 1]  RotationSequenceAxes=FollowerAxes  RotationSequence=XYX  RotationSequenceAngles=[0 0 0]  RotationSequenceAnglesUnits=deg  RotationMatrix=[1 0 0;0 1 0;0 0 1]  Quaternion=[1 0 0 0]  TranslationMethod=StandardAxis  TranslationCartesianOffset=[0 0 0]  TranslationCartesianOffsetUnits=m  TranslationStandardAxis=-Z  TranslationStandardOffset=0.005  TranslationStandardOffsetUnits=m  TranslationROffset=0  TranslationROffsetUnits=m  TranslationThetaOffset=0  TranslationThetaOffsetUnits=deg  TranslationZOffset=0  TranslationZOffsetUnits=m
  Rigid Transform1 : sm_lib/Frames and Transforms/Rigid Transform  RotationMethod=None  FollAlignAxisA=+X  BaseAlignAxisA=+Y  FollAlignAxisB=+Y  BaseAlignAxisB=+Z  RotationStandardAxis=+Z  RotationAngle=0  RotationAngleUnits=deg  RotationArbitraryAxis=[0 0 1]  RotationSequenceAxes=FollowerAxes  RotationSequence=XYX  RotationSequenceAngles=[0 0 0]  RotationSequenceAnglesUnits=deg  RotationMatrix=[1 0 0;0 1 0;0 0 1]  Quaternion=[1 0 0 0]  TranslationMethod=StandardAxis  TranslationCartesianOffset=[0 0 0]  TranslationCartesianOffsetUnits=m  TranslationStandardAxis=+Z  TranslationStandardOffset=0.5+0.2  TranslationStandardOffsetUnits=m  TranslationROffset=0  TranslationROffsetUnits=m  TranslationThetaOffset=0  TranslationThetaOffsetUnits=deg  TranslationZOffset=0  TranslationZOffsetUnits=m
  Rigid Transform6 : sm_lib/Frames and Transforms/Rigid Transform  RotationMethod=None  FollAlignAxisA=+X  BaseAlignAxisA=+Y  FollAlignAxisB=+Y  BaseAlignAxisB=+Z  RotationStandardAxis=+Y  RotationAngle=90  RotationAngleUnits=deg  RotationArbitraryAxis=[0 0 1]  RotationSequenceAxes=FollowerAxes  RotationSequence=XYX  RotationSequenceAngles=[0 0 0]  RotationSequenceAnglesUnits=deg  RotationMatrix=[0 0 1; 0 1 0; 1 0 0]  Quaternion=[1 0 0 0]  TranslationMethod=StandardAxis  TranslationCartesianOffset=[0 0 0]  TranslationCartesianOffsetUnits=m  TranslationStandardAxis=+Z  TranslationStandardOffset=1  TranslationStandardOffsetUnits=m  TranslationROffset=0  TranslationROffsetUnits=m  TranslationThetaOffset=0  TranslationThetaOffsetUnits=deg  TranslationZOffset=0  TranslationZOffsetUnits=m
  Scope{,1..2,4} (4 alike) : Scope
      Scope settings: ActiveDisplayYMinimum=-2.0138256178390441  ActiveDisplayYMaximum=0.22375840215241163  DataLoggingVariableName=ScopeData14
      Scope1 settings: ActiveDisplayYMinimum=-1.7669526132397224  ActiveDisplayYMaximum=0.19632806813774689  DataLoggingVariableName=ScopeData15
      Scope2 settings: ActiveDisplayYMinimum=-1  ActiveDisplayYMaximum=1  DataLoggingVariableName=ScopeData16
      Scope4 settings: ActiveDisplayYMinimum=-3.5002430122464903  ActiveDisplayYMaximum=3.7161890846826382  DataLoggingVariableName=ScopeData18
  Simulink-PS Converter1 : nesl_utility/Simulink-PS Converter  PhysicalDomain=network_engine_domain  SubClassName=ps_input  LeftPortType=input  RightPortType=output  PseudoPeriodic=off  Frequencies=[]  NoiseDistribution=none  NoiseParameters=[]  Unit=1  AffineConversion=off  FilteringAndDerivatives=zero  SimscapeFilterOrder=1  InputFilterTimeConstant=0.001  UdotUserProvided=1
  Simulink-PS Converter3 : nesl_utility/Simulink-PS Converter  PhysicalDomain=network_engine_domain  SubClassName=ps_input  LeftPortType=input  RightPortType=output  PseudoPeriodic=off  Frequencies=[]  NoiseDistribution=none  NoiseParameters=[]  Unit=1  AffineConversion=off  FilteringAndDerivatives=zero  SimscapeFilterOrder=1  InputFilterTimeConstant=0.001  UdotUserProvided=1
  Simulink-PS Converter4 : nesl_utility/Simulink-PS Converter  PhysicalDomain=network_engine_domain  SubClassName=ps_input  LeftPortType=input  RightPortType=output  PseudoPeriodic=off  Frequencies=[]  NoiseDistribution=none  NoiseParameters=[]  Unit=1  AffineConversion=off  FilteringAndDerivatives=zero  SimscapeFilterOrder=1  InputFilterTimeConstant=0.001  UdotUserProvided=1
  Solver Configuration : nesl_utility/Solver Configuration  PhysicalDomain=network_engine_domain  SubClassName=solver  LeftPortType=input  RightPortType=generic  Tones=[]  Harmonics=[]  SimulateNoise=off  Profile=off  UseLocalSampling=off  EnableSwitchedLinearOptims=on  FrequencyDomain=off  UseCCode=off  RelTol=0.001  AbsTol=1e-06  MinStep=1e-09  ToWorkspace=off  RevertToSquareIcSolve=off  NumHomotopyIterations=100  PhasorMode=off  PhasorModeNumHarmonics=1  ConsistencySolver=NEWTON_FTOL  IndexReductionMethod=DerivativeReplacement  DoDC=off  ResidualTolerance=1e-09  ConsistencyTolSource=GLOBAL  ConsistencyAbsTol=0.001  ConsistencyRelTol=0.001  ConsistencyTolFactor=0.001  UseLocalSolver=off  LocalSolverChoice=NE_BACKWARD_EULER_ADVANCER  ResolveIndetEquations=on  FunctionEvalNumThread=1  LocalSolverSampleTime=0.001  DoFixedCost=off  MaxNonlinIter=3  MaxModeIter=2  ComputeImpulses=off  ImpulseIterations=2  LinearAlgebra=Sparse  LinearAlgebraNumThread=0  EquationFormulation=NE_TIME_EF  DelaysMemoryBudget=1024  AutomaticFiltering=on  FilteringTimeConstant=0.001  PartitionStorageMethod=AS_NEEDED  PartitionMemoryBudget=1024  PartitionMethod=FAST  MultibodyUseLocalSolver=off  MultibodyLocalSolverChoice=ODE1  MultibodyLocalSolverSampleTime=0.001
  Spatial Contact Force1 : sm_lib/Forces and Torques/Spatial Contact Force  SenseSeparationDistance=off  NormalForceType=SmoothSpringDamper  NormalStiffness=1e6  NormalStiffnessUnits=N/m  NormalDamping=1e3  NormalDampingUnits=N/(m/s)  NormalTransitionRegionWidth=1e-4  NormalTransitionRegionWidthUnits=m  FrictionType=SmoothStickSlip  CoefficientOfStaticFriction=1  CoefficientOfDynamicFriction=1  FrictionalCriticalVelocity=1  FrictionalCriticalVelocityUnits=m/s  SenseContactSignal=off  SensePenetrationDepth=off  SenseNormalVelocity=off  SenseTangentialVelocity=off  SensingForceTorqueDirection=BaseOnFollower  SensingForceTorqueResolutionFrame=ContactFrame  SenseNormalForce=off  SenseNormalForceMagnitude=off  SenseNormalTorque=off  SenseFrictionalForce=off  SenseFrictionalForceMagnitude=off  SenseFrictionalTorque=off  SenseTotalForce=off  SenseTotalTorque=off  SenseContactBaseRotation=off  SenseContactBaseTranslation=off  SenseContactFollowerRotation=off  SenseContactFollowerTranslation=off  ZeroCrossDetectContactStartAndEnd=off
  Spatial Contact Force2 : sm_lib/Forces and Torques/Spatial Contact Force  SenseSeparationDistance=off  NormalForceType=SmoothSpringDamper  NormalStiffness=1e6  NormalStiffnessUnits=N/m  NormalDamping=1e3  NormalDampingUnits=N/(m/s)  NormalTransitionRegionWidth=1e-4  NormalTransitionRegionWidthUnits=m  FrictionType=SmoothStickSlip  CoefficientOfStaticFriction=0.5  CoefficientOfDynamicFriction=0.3  FrictionalCriticalVelocity=1e-3  FrictionalCriticalVelocityUnits=m/s  SenseContactSignal=off  SensePenetrationDepth=off  SenseNormalVelocity=off  SenseTangentialVelocity=off  SensingForceTorqueDirection=BaseOnFollower  SensingForceTorqueResolutionFrame=ContactFrame  SenseNormalForce=off  SenseNormalForceMagnitude=off  SenseNormalTorque=off  SenseFrictionalForce=off  SenseFrictionalForceMagnitude=off  SenseFrictionalTorque=off  SenseTotalForce=off  SenseTotalTorque=off  SenseContactBaseRotation=off  SenseContactBaseTranslation=off  SenseContactFollowerRotation=off  SenseContactFollowerTranslation=off  ZeroCrossDetectContactStartAndEnd=off
  Spatial Contact Force3 : sm_lib/Forces and Torques/Spatial Contact Force  SenseSeparationDistance=off  NormalForceType=SmoothSpringDamper  NormalStiffness=1e6  NormalStiffnessUnits=N/m  NormalDamping=1e3  NormalDampingUnits=N/(m/s)  NormalTransitionRegionWidth=1e-4  NormalTransitionRegionWidthUnits=m  FrictionType=SmoothStickSlip  CoefficientOfStaticFriction=1  CoefficientOfDynamicFriction=1  FrictionalCriticalVelocity=1  FrictionalCriticalVelocityUnits=m/s  SenseContactSignal=off  SensePenetrationDepth=off  SenseNormalVelocity=off  SenseTangentialVelocity=off  SensingForceTorqueDirection=BaseOnFollower  SensingForceTorqueResolutionFrame=ContactFrame  SenseNormalForce=off  SenseNormalForceMagnitude=off  SenseNormalTorque=off  SenseFrictionalForce=off  SenseFrictionalForceMagnitude=off  SenseFrictionalTorque=off  SenseTotalForce=off  SenseTotalTorque=off  SenseContactBaseRotation=off  SenseContactBaseTranslation=off  SenseContactFollowerRotation=off  SenseContactFollowerTranslation=off  ZeroCrossDetectContactStartAndEnd=off
  Spherical Solid : sm_lib/Body Elements/Spherical Solid  Commented=on  SphereRadius=0.1  SphereRadiusUnits=m  ExportEntireGeometry=off  InertiaType=CalculateFromGeometry  BasedOnType=Density  Density=1000  DensityUnits=kg/m^3  Mass=6  MassUnits=kg  CenterOfMass=[0 0 0]  CenterOfMassUnits=m  MomentsOfInertia=[1 1 1]  MomentsOfInertiaUnits=kg*m^2  ProductsOfInertia=[0 0 0]  ProductsOfInertiaUnits=kg*m^2  GraphicType=FromGeometry  MarkerShape=Sphere  MarkerSize=10  GraphicVisPropType=AdvancedVisualProperties  GraphicDiffuseColor=[0.5 0.5 0.5]  GraphicOpacity=1  GraphicSpecularColor=[0.8275 0.8275 0.8275]  GraphicAmbientColor=[0.15 0.15 0.15 1.0]  GraphicEmissiveColor=[0.0 0.0 0.0 1.0]  GraphicShininess=75  DoExposeReferenceFrame=on  SerializedFrames=<Frames/>
  Transform Sensor : sm_lib/Frames and Transforms/Transform Sensor  MeasurementFrame=World  RotationSequence=ZYX  SenseAngle=off  SenseAxis=off  SenseQ=off  SenseR=off  SenseRotationSequence=on  SenseOmegaX=off  SenseOmegaY=off  SenseOmegaZ=off  SenseOmega=off  SenseQDot=off  SenseRDot=off  SenseRotationSequenceDot=off  SenseAlphaX=off  SenseAlphaY=off  SenseAlphaZ=off  SenseAlpha=off  SenseQDDot=off  SenseRDDot=off  SenseX=off  SenseY=off  SenseZ=off  SenseXYZ=off  SenseRad=off  SenseAzim=off  SenseDist=off  SenseInc=off  SenseXDot=off  SenseYDot=off  SenseZDot=off  SenseXYZDot=off  SenseRadDot=off  SenseAzimDot=off  SenseDistDot=off  SenseIncDot=off  SenseXDDot=off  SenseYDDot=off  SenseZDDot=off  SenseXYZDDot=off  SenseRadDDot=off  SenseAzimDDot=off  SenseDistDDot=off  SenseIncDDot=off
  Transform lw : sm_lib/Frames and Transforms/Rigid Transform  RotationMethod=StandardAxis  FollAlignAxisA=+X  BaseAlignAxisA=+Y  FollAlignAxisB=+Y  BaseAlignAxisB=+Z  RotationStandardAxis=-X  RotationAngle=90  RotationAngleUnits=deg  RotationArbitraryAxis=[0 0 1]  RotationSequenceAxes=FollowerAxes  RotationSequence=XYX  RotationSequenceAngles=[0 0 0]  RotationSequenceAnglesUnits=deg  RotationMatrix=[1 0 0; 0 1 0; 0 0 1]  Quaternion=[1 0 0 0]  TranslationMethod=StandardAxis  TranslationCartesianOffset=[0 0 0]  TranslationCartesianOffsetUnits=m  TranslationStandardAxis=+Y  TranslationStandardOffset=ly/2+t/2  TranslationStandardOffsetUnits=m  TranslationROffset=0  TranslationROffsetUnits=m  TranslationThetaOffset=0  TranslationThetaOffsetUnits=deg  TranslationZOffset=0  TranslationZOffsetUnits=m
  Transform rw1 : sm_lib/Frames and Transforms/Rigid Transform  RotationMethod=StandardAxis  FollAlignAxisA=+X  BaseAlignAxisA=+Y  FollAlignAxisB=+Y  BaseAlignAxisB=+Z  RotationStandardAxis=-X  RotationAngle=90  RotationAngleUnits=deg  RotationArbitraryAxis=[0 0 1]  RotationSequenceAxes=FollowerAxes  RotationSequence=XYX  RotationSequenceAngles=[0 0 0]  RotationSequenceAnglesUnits=deg  RotationMatrix=[1 0 0; 0 1 0; 0 0 1]  Quaternion=[1 0 0 0]  TranslationMethod=StandardAxis  TranslationCartesianOffset=[0 0 0]  TranslationCartesianOffsetUnits=m  TranslationStandardAxis=-Y  TranslationStandardOffset=ly/2+t/2  TranslationStandardOffsetUnits=m  TranslationROffset=0  TranslationROffsetUnits=m  TranslationThetaOffset=0  TranslationThetaOffsetUnits=deg  TranslationZOffset=0  TranslationZOffsetUnits=m
  World Frame : sm_lib/Frames and Transforms/World Frame
  leftWheel : sm_lib/Body Elements/Cylindrical Solid  CylinderRadius=r  CylinderRadiusUnits=m  CylinderLength=t  CylinderLengthUnits=m  ExportEntireGeometry=on  InertiaType=CalculateFromGeometry  BasedOnType=Mass  Density=1000  DensityUnits=kg/m^3  Mass=m_w  MassUnits=kg  CenterOfMass=[0 0 0]  CenterOfMassUnits=m  MomentsOfInertia=[1 1 1]  MomentsOfInertiaUnits=kg*m^2  ProductsOfInertia=[0 0 0]  ProductsOfInertiaUnits=kg*m^2  GraphicType=FromGeometry  MarkerShape=Sphere  MarkerSize=10  GraphicVisPropType=SimpleVisualProperties  GraphicDiffuseColor=[0.5 0.5 0.5]  GraphicOpacity=1  GraphicSpecularColor=[0.5 0.5 0.5 1.0]  GraphicAmbientColor=[0.15 0.15 0.15 1.0]  GraphicEmissiveColor=[0.0 0.0 0.0 1.0]  GraphicShininess=75  DoExposeReferenceFrame=on  SerializedFrames=<Frames/>
  rightWheel : sm_lib/Body Elements/Cylindrical Solid  CylinderRadius=r  CylinderRadiusUnits=m  CylinderLength=t  CylinderLengthUnits=m  ExportEntireGeometry=on  InertiaType=CalculateFromGeometry  BasedOnType=Mass  Density=1000  DensityUnits=kg/m^3  Mass=m_w  MassUnits=kg  CenterOfMass=[0 0 0]  CenterOfMassUnits=m  MomentsOfInertia=[1 1 1]  MomentsOfInertiaUnits=kg*m^2  ProductsOfInertia=[0 0 0]  ProductsOfInertiaUnits=kg*m^2  GraphicType=FromGeometry  MarkerShape=Sphere  MarkerSize=10  GraphicVisPropType=SimpleVisualProperties  GraphicDiffuseColor=[0.5 0.5 0.5]  GraphicOpacity=1  GraphicSpecularColor=[0.5 0.5 0.5 1.0]  GraphicAmbientColor=[0.15 0.15 0.15 1.0]  GraphicEmissiveColor=[0.0 0.0 0.0 1.0]  GraphicShininess=75  DoExposeReferenceFrame=on  SerializedFrames=<Frames/>
  rw_angle : Outport  VectorParamsAs1DForOutWhenUnconnected=off
  lw_angle : Outport  Port=2  VectorParamsAs1DForOutWhenUnconnected=off
  pitch_angle : Outport  Port=3  VectorParamsAs1DForOutWhenUnconnected=off
  wires:
  PS-Simulink Converter1/1 -> rw_angle/1
  dF/1 -> Simulink-PS Converter1/1
  PS-Simulink Converter2/1 -> lw_angle/1
  rwTorque/1 -> Simulink-PS Converter3/1
  PS-Simulink Converter4/1 -> Demux/1, Scope4/1
  Demux/2 -> Scope1/1, pitch_angle/1  "pitch"
  Demux/3 -> Scope2/1  "roll"
  Demux/1 -> Scope/1  "yaw"
  lwTorque/1 -> Simulink-PS Converter4/1
  connections:
  World Frame/RConn1 -- Solver Configuration/RConn1 -- Rigid Transform1/LConn1 -- Rigid Transform/LConn1 -- Mechanism Configuration/RConn1 -- Transform Sensor/LConn1
  Simulink-PS Converter1/RConn1 -- External Force and Torque/LConn1
  External Force and Torque/RConn1 -- Spherical Solid/RConn1 -- Rigid Transform6/RConn1
  Rigid Transform/RConn1 -- Floor/RConn1
  Spatial Contact Force3/LConn1 -- Spatial Contact Force1/LConn1 -- Spatial Contact Force2/LConn1 -- Floor/LConn1
  rightWheel/LConn1 -- Spatial Contact Force3/RConn1
  Transform rw1/RConn1 -- Revolute rw/LConn1
  Revolute rw/RConn1 -- rightWheel/RConn1
  Brick/LConn1 -- Rigid Transform6/LConn1 -- Transform Sensor/RConn1 -- Transform lw/LConn1 -- Transform rw1/LConn1
  Revolute lw/RConn1 -- leftWheel/RConn1
  Transform lw/RConn1 -- Revolute lw/LConn1
  Spatial Contact Force1/RConn1 -- leftWheel/LConn1
  Revolute rw/LConn2 -- Simulink-PS Converter3/RConn1
  Revolute lw/LConn2 -- Simulink-PS Converter4/RConn1
  Spatial Contact Force2/RConn1 -- Brick/LConn2
  6-DOF Joint/LConn1 -- Rigid Transform1/RConn1
  6-DOF Joint/RConn1 -- Brick/RConn1
  Transform Sensor/RConn2 -- PS-Simulink Converter4/LConn1
  Revolute rw/RConn2 -- PS-Simulink Converter1/LConn1
  Revolute lw/RConn2 -- PS-Simulink Converter2/LConn1
